simulink model "RobotNARX"  (R2013a)
settings: Solver=ode45  StartTime=0.0  StopTime=n  RelTol=1e-3
values from neighbouring files (symbols this model uses):
  x0 = findstates(Model,[tXv in4v])    [Robot.m]
libraries: slident x2
settings Model: Creator=Saeed  LastModifiedBy=Saeed
settings DataIOCC: SignalLoggingSaveFormat=ModelDataLogs
settings OptimizationCC: ExpressionDepthLimit=2147483647
settings DebuggingCC: FcnCallInpInsideContextMsg=EnableAllAsWarning

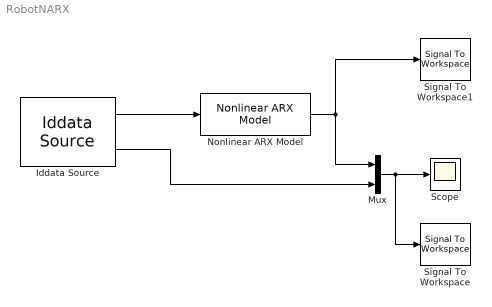
== system RobotNARX ==
  Iddata Source : slident/Iddata Source  iddataobj=XX
  Mux : Mux  Inputs=2
  Nonlinear ARX Model : slident/Nonlinear ARX Model  sys=Model  ICspec=State values  X0=x0  U0=init1  Y0=-0.055114518394625
  Scope : Scope
  Signal To Workspace : SignalToWorkspace  VariableName=yout  SaveFormat=Timeseries
      settings: CopyFcn=dspblkcopystw(gcbh);
  Signal To Workspace1 : SignalToWorkspace  VariableName=mout
      settings: CopyFcn=dspblkcopystw(gcbh);
  wires:
  Iddata Source/1 -> Nonlinear ARX Model/1
  Nonlinear ARX Model/1 -> Mux/1, Signal To Workspace1/1
  Mux/1 -> Scope/1, Signal To Workspace/1
  Iddata Source/2 -> Mux/2
